simulink model "quadcopter_sim"  (R2023a)
settings: Solver=ode4  StartTime=0.0  StopTime=t_lim  FixedStep=t_s  RelTol=1e-3
InitFcn:
  | init_quadcopter
values from neighbouring files (symbols this model uses):
  C_CCW = [-C(1), C(2)]    [init_quadcopter.m]
  C_CW = [ C(1), C(2)]    [init_quadcopter.m]
  RP1 = [ dims(1)/2,  dims(2)/2, dims(3)/2]'    [init_quadcopter.m]
  RP2 = [-dims(1)/2,  dims(2)/2, dims(3)/2]'    [init_quadcopter.m]
  RP3 = [-dims(1)/2, -dims(2)/2, dims(3)/2]'    [init_quadcopter.m]
  RP4 = [ dims(1)/2, -dims(2)/2, dims(3)/2]'    [init_quadcopter.m]
  V = zeros(3,t_lim/t_s)    [init_quadcopter.m]
  W = zeros(3,t_lim/t_s)    [init_quadcopter.m]
  X = zeros(3,t_lim/t_s)    [init_quadcopter.m]
undefined symbols (not defined in the file or in its folder): quadcopter
libraries: matrix_library x4, shared6dof x1
settings Model: Creator=Bugra  LastModifiedBy=Bugra

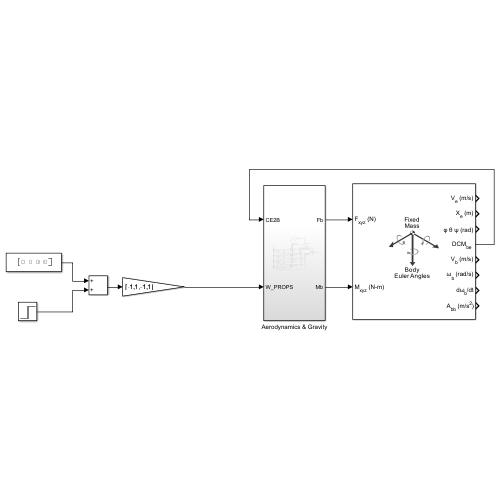
[thumbnail: Simulink's stored preview of the top-level diagram]
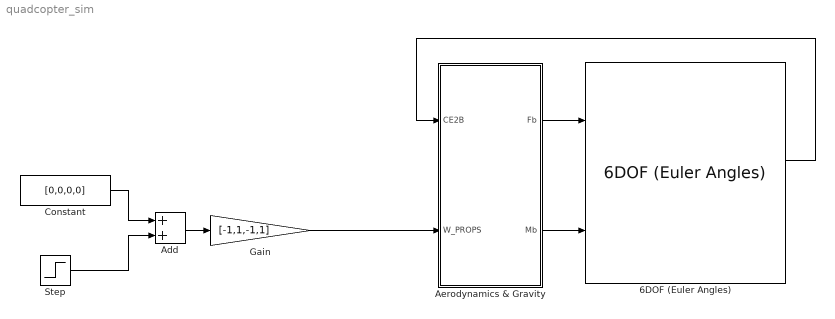
== system quadcopter_sim ==
  6DOF (Euler Angles) : shared6dof/6DOF (Euler Angles)  units=Metric (MKS)  mtype=Fixed  rep=Euler Angles  xme_0=X(:,1)'  Vm_0=V(:,1)'  eul_0=E(:,1)'  pm_0=W(:,1)'  mass_0=quadcopter.m  mass_e=0.5  mass_f=2.0  inertia=quadcopter.j  inertia_e=eye(3)  inertia_f=2*eye(3)  k_quat=1.0  vre_flag=on  abi_flag=off  aMode=0  xme_statename=''  Vm_statename=''  eul_statename=''  quat_statename=''  pm_statename=''  mass_statename=''
  Add : Sum
  Aerodynamics & Gravity : Subsystem
  Constant : Constant  Value=[0,0,0,0]
  Gain : Gain  Gain=[-1,1,-1,1]
  Step : Step  Time=0  After=186  SampleTime=0
  wires:
  Aerodynamics & Gravity/1(Fb) -> 6DOF (Euler Angles)/1
  6DOF (Euler Angles)/4 -> Aerodynamics & Gravity/1(CE2B)
  Aerodynamics & Gravity/2(Mb) -> 6DOF (Euler Angles)/2
  Step/1 -> Add/2
  Constant/1 -> Add/1
  Add/1 -> Gain/1
  Gain/1 -> Aerodynamics & Gravity/2(W_PROPS)

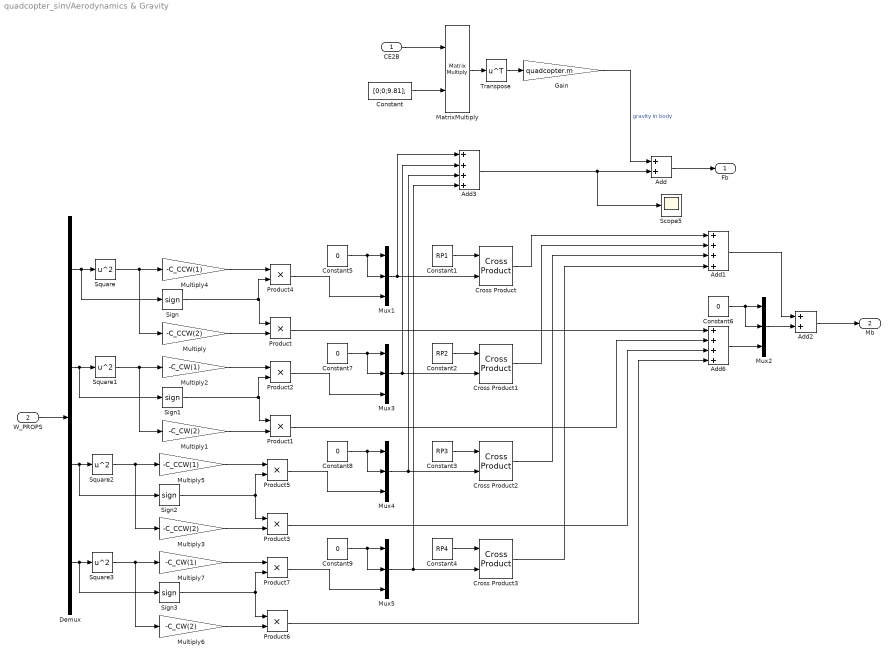
== system quadcopter_sim/Aerodynamics & Gravity ==
  CE2B : Inport
  W_PROPS : Inport  Port=2
  Add : Sum
  Add1 : Sum  Inputs=++++
  Add2 : Sum
  Add3 : Sum  Inputs=++++
  Add6 : Sum  Inputs=++++
  Constant : Constant  Value=[0;0;9.81];
  Constant1 : Constant  Value=RP1
  Constant2 : Constant  Value=RP2
  Constant3 : Constant  Value=RP3
  Constant4 : Constant  Value=RP4
  Constant{5..9} (5 alike) : Constant  Value=0
  Cross Product{,1..3} (4 alike) : matrix_library/Cross Product
  Demux : Demux
  Gain : Gain  Gain=quadcopter.m
  MatrixMultiply : Product  Multiplication=Matrix(*)
  Multiply : Gain  Gain=-C_CCW(2)
  Multiply1 : Gain  Gain=-C_CW(2)
  Multiply2 : Gain  Gain=-C_CW(1)
  Multiply3 : Gain  Gain=-C_CCW(2)
  Multiply4 : Gain  Gain=-C_CCW(1)
  Multiply5 : Gain  Gain=-C_CCW(1)
  Multiply6 : Gain  Gain=-C_CW(2)
  Multiply7 : Gain  Gain=-C_CW(1)
  Mux{1..5} (5 alike) : Mux  Inputs=3
  Product{,1..7} (8 alike) : Product
  Scope5 : Scope
  Sign{,1..3} (4 alike) : Signum
  Square{,1..3} (4 alike) : Math  Operator=square
  Transpose : Math  Operator=transpose
  Fb : Outport
  Mb : Outport  Port=2
  wires:
  Add/1 -> Fb/1
  CE2B/1 -> MatrixMultiply/1
  Constant/1 -> MatrixMultiply/2
  MatrixMultiply/1 -> Transpose/1
  Transpose/1 -> Gain/1
  W_PROPS/1 -> Demux/1
  Add2/1 -> Mb/1
  Constant1/1 -> Cross Product/1
  Demux/1 -> Sign/1, Square/1
  Sign/1 -> Product4/2, Product/1
  Multiply/1 -> Product/2
  Square/1 -> Multiply/1, Multiply4/1
  Multiply4/1 -> Product4/1
  Cross Product/1 -> Add1/1
  Product/1 -> Add6/1
  Square1/1 -> Multiply1/1, Multiply2/1
  Sign1/1 -> Product2/2, Product1/1
  Multiply2/1 -> Product2/1
  Multiply1/1 -> Product1/2
  Constant2/1 -> Cross Product1/1
  Demux/2 -> Sign1/1, Square1/1
  Cross Product1/1 -> Add1/2
  Product1/1 -> Add6/2
  Product3/1 -> Add6/3
  Square2/1 -> Multiply3/1, Multiply5/1
  Sign2/1 -> Product5/2, Product3/1
  Multiply5/1 -> Product5/1
  Multiply3/1 -> Product3/2
  Constant3/1 -> Cross Product2/1
  Demux/3 -> Sign2/1, Square2/1
  Cross Product2/1 -> Add1/3
  Product6/1 -> Add6/4
  Square3/1 -> Multiply6/1, Multiply7/1
  Sign3/1 -> Product7/2, Product6/1
  Multiply7/1 -> Product7/1
  Multiply6/1 -> Product6/2
  Constant4/1 -> Cross Product3/1
  Demux/4 -> Sign3/1, Square3/1
  Cross Product3/1 -> Add1/4
  Constant5/1 -> Mux1/2, Mux1/1
  Constant6/1 -> Mux2/1, Mux2/2
  Add6/1 -> Mux2/3
  Mux1/1 -> Add3/1, Cross Product/2
  Mux3/1 -> Cross Product1/2, Add3/2
  Product2/1 -> Mux3/3
  Constant7/1 -> Mux3/2, Mux3/1
  Product5/1 -> Mux4/3
  Constant8/1 -> Mux4/2, Mux4/1
  Mux4/1 -> Cross Product2/2, Add3/3
  Product7/1 -> Mux5/3
  Constant9/1 -> Mux5/2, Mux5/1
  Mux5/1 -> Cross Product3/2, Add3/4
  Mux2/1 -> Add2/2
  Add1/1 -> Add2/1
  Add3/1 -> Scope5/1, Add/2
  Product4/1 -> Mux1/3
  Gain/1 -> Add/1  "gravity in body"
